simulink subsystem "decoder"  (R2022b)
settings: Solver=VariableStepAuto  StartTime=0.0  StopTime=10.0  RelTol=1e-3
settings Model: Creator=LeonK  LastModifiedBy=LeonK

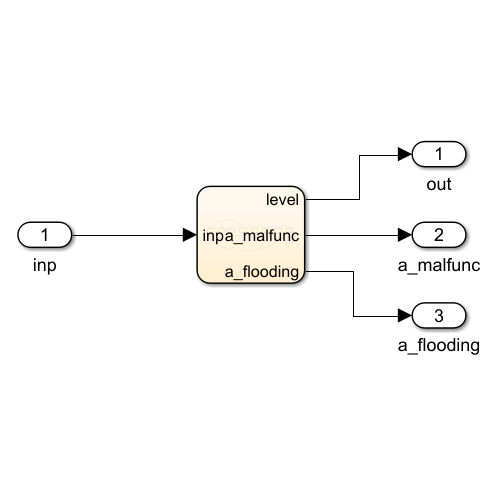
[thumbnail: Simulink's stored preview of the top-level diagram]
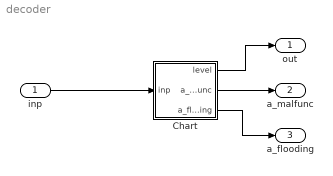
== system decoder ==
  inp : Inport
  Chart : Stateflow chart  TreatAsAtomicUnit=on
  out : Outport
  a_malfunc : Outport  Port=2
  a_flooding : Outport  Port=3
  wires:
  Chart/3(a_flooding) -> a_flooding/1
  Chart/2(a_malfunc) -> a_malfunc/1
  Chart/1(level) -> out/1
  inp/1 -> Chart/1(inp)

== stateflow chart decoder/Chart ==
  state q0
    a_malfunc=0;
    a_flooding=0;
  state q_malfunction
    level=1;
    a_malfunc=1;
  state q01
    level=1;
  state q_0_10
    level=2;
  state q_10_20
    level=3;
  state q_20_30
    level=4;
  state q_30_max
    level=5;
  state q_overflow
    level=5;
    a_flooding=1;
  q0 -> q01 [order 1] : [inp==0]
  q_malfunction -> q_malfunction : [inp==0 || inp==1]
  q01 -> q_0_10 [order 2] : [inp==1]
  q_30_max -> q_overflow [order 1] : [inp==1]
  q_20_30 -> q_30_max [order 1] : [inp==1]
  q_0_10 -> q_10_20 [order 1] : [inp==1]
  (default) -> q0
  q_10_20 -> q_20_30 [order 1] : [inp==1]
  q0 -> q_30_max [order 2] : [inp==1]
  q01 -> q_malfunction [order 1] : [inp==0]
  q_0_10 -> q01 [order 2] : [inp==0]
  q_10_20 -> q_0_10 [order 2] : [inp==0]
  q_20_30 -> q_10_20 [order 2] : [inp==0]
  q_30_max -> q_20_30 [order 2] : [inp==0]
  q_overflow -> q_overflow : [inp==0 || inp==1]
  data: inp input; level output; a_malfunc output; a_flooding output
